simulink model "seguidor_primero"  (R2019a)
settings: Solver=VariableStepAuto  StartTime=0.0  StopTime=20  RelTol=1e-3
values from neighbouring files (symbols this model uses):
  ki = ka(1:end,m+1:end)    [programa_seguidor.m]
  kp = ka(1:end,1:m)    [programa_seguidor.m]
undefined symbols (not defined in the file or in its folder): A2, B2, C2
settings Model: Creator=Alejoxbg  LastModifiedBy=Alejoxbg

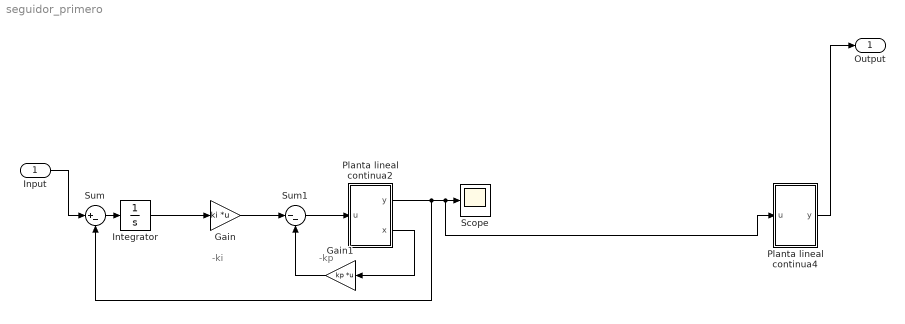
== system seguidor_primero ==
  note: -ki
  note: -kp
  Input : Inport
  Gain : Gain  Gain=ki  Multiplication=Matrix(K*u) (u vector)
  Gain1 : Gain  Gain=kp  Multiplication=Matrix(K*u) (u vector)
  Integrator : Integrator
  Planta lineal continua2 : Subsystem
  Planta lineal continua4 : Subsystem
  Scope : Scope
  Sum : Sum  Inputs=|+-
  Sum1 : Sum  Inputs=|--
  Output : Outport
  wires:
  Input/1 -> Sum/1
  Sum/1 -> Integrator/1
  Integrator/1 -> Gain/1
  Planta lineal continua2/1(y) -> Planta lineal continua4/1(u), Scope/1, Sum/2
  Gain/1 -> Sum1/1
  Gain1/1 -> Sum1/2
  Sum1/1 -> Planta lineal continua2/1(u)
  Planta lineal continua2/2(x) -> Gain1/1
  Planta lineal continua4/1(y) -> Output/1

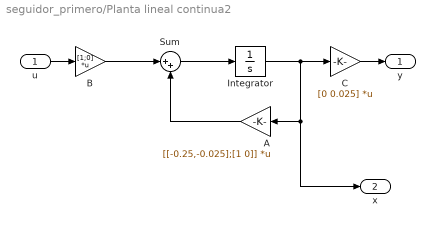
== system seguidor_primero/Planta lineal continua2 ==
  u : Inport
  A : Gain  Gain=[[-0.25,-0.025];[1 0]]  Multiplication=Matrix(K*u) (u vector)
  B : Gain  Gain=[1;0]  Multiplication=Matrix(K*u) (u vector)
  C : Gain  Gain=[0 0.025]  Multiplication=Matrix(K*u) (u vector)
  Integrator : Integrator
  Sum : Sum  Inputs=|++
  y : Outport
  x : Outport  Port=2
  wires:
  C/1 -> y/1
  u/1 -> B/1
  Integrator/1 -> x/1, A/1, C/1
  A/1 -> Sum/2
  Sum/1 -> Integrator/1
  B/1 -> Sum/1

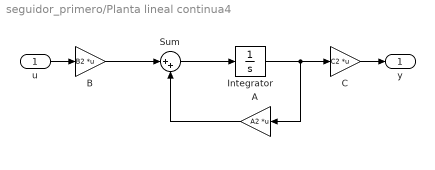
== system seguidor_primero/Planta lineal continua4 ==
  u : Inport
  A : Gain  Gain=A2  Multiplication=Matrix(K*u) (u vector)
  B : Gain  Gain=B2  Multiplication=Matrix(K*u) (u vector)
  C : Gain  Gain=C2  Multiplication=Matrix(K*u) (u vector)
  Integrator : Integrator
  Sum : Sum  Inputs=|++
  y : Outport
  wires:
  C/1 -> y/1
  u/1 -> B/1
  Integrator/1 -> A/1, C/1
  A/1 -> Sum/2
  Sum/1 -> Integrator/1
  B/1 -> Sum/1
